simulink model "MalaksModel"  (R2022a)
settings: Solver=FixedStepAuto  StartTime=0.0  StopTime=10  FixedStep=0.001  MaxStep=1  MinStep=5e-4  RelTol=1e-3  EnableMultiTasking=on
values from neighbouring files (symbols this model uses):
  B = 0.00416    [Allan_Param.m]
  b1 = Bf/2    (= 0.776)    [model_10DOF_revised.m]
  b2 = b1    (= 0.776)    [model_10DOF_revised.m]
  b3 = Br/2    (= 0.78)    [model_10DOF_revised.m]
  b4 = b3    (= 0.78)    [model_10DOF_revised.m]
  Beq = 0.0001    [model_10DOF_revised.m]
  Bf = 1.552    [model_10DOF_revised.m]
  cs1 = 4500    [model_10DOF_revised.m]
  cs2 = 4500    [model_10DOF_revised.m]
  cs3 = 11207    [model_10DOF_revised.m]
  dpc = h-hzpc    (= 0.4878144918)    [model_10DOF_revised.m]
  drc = h-hzrc    (= 0.4878144918)    [model_10DOF_revised.m]
  Fs = 100    [Allan_Param.m]
  g = 9.81    [model_10DOF_revised.m]
  hzpc = 0.05    [model_10DOF_revised.m]
  hzrc = 0.05    [model_10DOF_revised.m]
  Ix = 233.072773102 + m*drc^2    (= 616.009936849)    [model_10DOF_revised.m]
  Ix_Iy = Ix -Iy    (= -852.927226898)    [model_10DOF_revised.m]
  Iy = 1086 + m*dpc^2    (= 1468.93716375)    [model_10DOF_revised.m]
  Iy_Iz = Iy -Iz    (= 281.937163747)    [model_10DOF_revised.m]
  Iz = 1187    [model_10DOF_revised.m]
  Iz_Ix = Iz -Ix    (= 570.990063151)    [model_10DOF_revised.m]
  Jeq = 0.00025    [model_10DOF_revised.m]
  K = 1.4e-3    (= 0.0014)    [Allan_Param.m]
  Ka = 0.05    [model_10DOF_revised.m]
  Ke = 0.168    [model_10DOF_revised.m]
  L = 2.72    [model_10DOF_revised.m]
  l1 = 1.12695753    [model_10DOF_revised.m]
  l2 = L-l1    (= 1.59304247)    [model_10DOF_revised.m]
  Leq = 1.5e-3    (= 0.0015)    [model_10DOF_revised.m]
  m = MT-(muf+mur)    (= 1609.23)    [model_10DOF_revised.m]
  mu = 0.8    [model_10DOF_revised.m]
  mu1 = muf/2    (= 49.5)    [model_10DOF_revised.m]
  mu2 = mu1    (= 49.5)    [model_10DOF_revised.m]
  mu3 = mur/2    (= 42)    [model_10DOF_revised.m]
  mu4 = mu3    (= 42)    [model_10DOF_revised.m]
  N = 0.00166667    [Allan_Param.m]
  radius = 40    [path1.m]
  Req = 0.5    [model_10DOF_revised.m]
  ro = 0    [Input.m]
  sw_delta_f = 1    [Input.m]
  Tc = 32    [Allan_Param.m]
  THETAo = 0    [Input.m]
  tpo = cp/6    (= 0.0333333333333)    [Input.m]
  vxo = 10    [Input.m]
  vyo = 0    [Input.m]
  Ws1 = (l2*Ws)/(2*L)    (= 4622.91152767)    [model_10DOF_revised.m]
  x = 0:1:200    [look_ahead.m]    (also in path1.m = x(:))
  Xo = 0    [Input.m]
  y = l_des    [look_ahead.m]    (also in path1.m = zeros(size(x)))
  Yo = 0    [Input.m]
  zu1_0 = -W1/k1t    (= -0.0255425326383)    [model_10DOF_revised.m]
  zu2_0 = -W2/k2t    (= -0.0255425326383)    [model_10DOF_revised.m]
  zu3_0 = -W3/k3t    (= -0.0184119081117)    [model_10DOF_revised.m]
  zu4_0 = -W4/k4t    (= -0.0184119081117)    [model_10DOF_revised.m]
undefined symbols (not defined in the file or in its folder): sw_phi, sw_psi, sw_theta, sw_x, sw_y, sw_zs, sw_zu1, sw_zu2, sw_zu3, sw_zu4
libraries: slpidlib x6, ec_arm_cortex_a_lib x1
(part 2 of 2)

== system MalaksModel/PID DC motor1/Ratchet ==
  d2 : Inport  OutDataTypeStr=double
  Memory3 : Memory
  Memory4 : Memory
  Ratchet : MATLAB Function  TreatAsAtomicUnit=on
  Switch : MATLAB Function  TreatAsAtomicUnit=on
  Theta : Outport  OutDataTypeStr=double
  wires:
  Memory3/1 -> Switch/2(d1)
  d2/1 -> Ratchet/1(d2), Switch/1(d2)
  Switch/2(d) -> Memory3/1
  Memory4/1 -> Ratchet/2(d1)
  Ratchet/1(y) -> Memory4/1, Theta/1  "Theta"
  Switch/1(y) -> Ratchet/3(s)

== system MalaksModel/PID DC motor2/Ratchet ==
  d2 : Inport  OutDataTypeStr=double
  Memory3 : Memory
  Memory4 : Memory
  Ratchet : MATLAB Function  TreatAsAtomicUnit=on
  Switch : MATLAB Function  TreatAsAtomicUnit=on
  Theta : Outport  OutDataTypeStr=double
  wires:
  Memory3/1 -> Switch/2(d1)
  d2/1 -> Ratchet/1(d2), Switch/1(d2)
  Switch/2(d) -> Memory3/1
  Memory4/1 -> Ratchet/2(d1)
  Ratchet/1(y) -> Memory4/1, Theta/1  "Theta"
  Switch/1(y) -> Ratchet/3(s)

== system MalaksModel/PID DC motor3/Ratchet ==
  d2 : Inport  OutDataTypeStr=double
  Memory3 : Memory
  Memory4 : Memory
  Ratchet : MATLAB Function  TreatAsAtomicUnit=on
  Switch : MATLAB Function  TreatAsAtomicUnit=on
  Theta : Outport  OutDataTypeStr=double
  wires:
  Memory3/1 -> Switch/2(d1)
  d2/1 -> Ratchet/1(d2), Switch/1(d2)
  Switch/2(d) -> Memory3/1
  Memory4/1 -> Ratchet/2(d1)
  Ratchet/1(y) -> Memory4/1, Theta/1  "Theta"
  Switch/1(y) -> Ratchet/3(s)

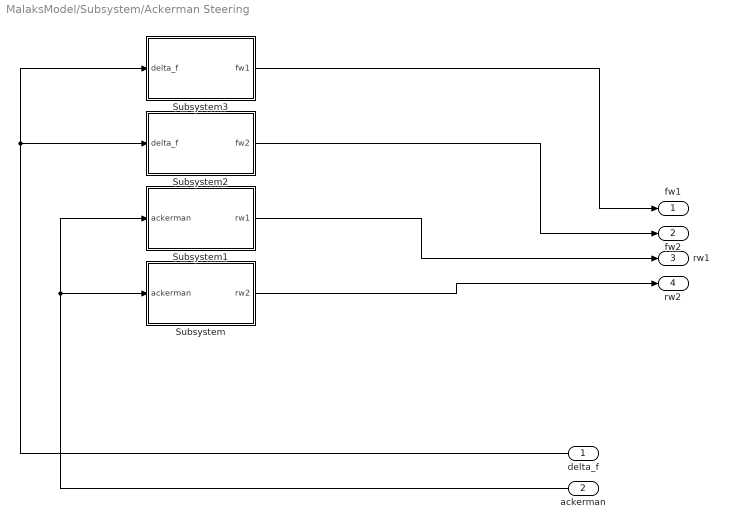
== system MalaksModel/Subsystem/Ackerman Steering ==
  delta_f : Inport  OutDataTypeStr=double
  ackerman : Inport  Port=2  OutDataTypeStr=double
  Subsystem : Subsystem
  Subsystem1 : Subsystem
  Subsystem2 : Subsystem
  Subsystem3 : Subsystem
  fw1 : Outport  OutDataTypeStr=double
  fw2 : Outport  Port=2  OutDataTypeStr=double
  rw1 : Outport  Port=3  OutDataTypeStr=double
  rw2 : Outport  Port=4  OutDataTypeStr=double
  wires:
  ackerman/1 -> Subsystem1/1(ackerman), Subsystem/1(ackerman)
  delta_f/1 -> Subsystem3/1(delta_f), Subsystem2/1(delta_f)
  Subsystem1/1(rw1) -> rw1/1
  Subsystem/1(rw2) -> rw2/1
  Subsystem3/1(fw1) -> fw1/1
  Subsystem2/1(fw2) -> fw2/1

== system MalaksModel/Subsystem/RWS ==
  delta_f : Inport  OutDataTypeStr=double
  vx : Inport  Port=2  OutDataTypeStr=double
  Constant : Constant  Value=l1
  Constant1 : Constant  Value=l2
  Constant2 : Constant  Value=L
  Constant3 : Constant  Value=m
  Constant4 : Constant  Value=cs3
  Constant5 : Constant  Value=cs2
  MATLAB Function : MATLAB Function  TreatAsAtomicUnit=on
  delta_r : Outport  OutDataTypeStr=double
  wires:
  Constant1/1 -> MATLAB Function/4(l2)
  vx/1 -> MATLAB Function/2(vx)
  Constant/1 -> MATLAB Function/3(l1)
  Constant3/1 -> MATLAB Function/6(m)
  Constant5/1 -> MATLAB Function/8(cs2)
  Constant2/1 -> MATLAB Function/5(L)
  Constant4/1 -> MATLAB Function/7(cs3)
  MATLAB Function/1(delta_r) -> delta_r/1
  delta_f/1 -> MATLAB Function/1(delta_f)

== system MalaksModel/Driver Steering Control/Subsystem/If Action Subsystem ==
  In1 : Inport
  Action Port : ActionPort  ActionPortLabel=if(u1 == 0)
  Out1 : Outport
  wires:
  In1/1 -> Out1/1

== system MalaksModel/Driver Steering Control/Subsystem/If Action Subsystem1 ==
  In1 : Inport
  Action Port : ActionPort  ActionPortLabel=elseif(u1 == 1)
  Out1 : Outport
  wires:
  In1/1 -> Out1/1

== system MalaksModel/Driver Steering Control/Subsystem1/If Action Subsystem ==
  In1 : Inport
  Action Port : ActionPort  ActionPortLabel=if(u1 == 0)
  Out1 : Outport
  wires:
  In1/1 -> Out1/1

== system MalaksModel/Driver Steering Control/Subsystem1/If Action Subsystem1 ==
  In1 : Inport
  Action Port : ActionPort  ActionPortLabel=elseif(u1 == 1)
  Out1 : Outport
  wires:
  In1/1 -> Out1/1

== system MalaksModel/Subsystem/Ackerman Steering/Subsystem ==
  ackerman : Inport
  Constant2 : Constant  Value=Bf
  Constant3 : Constant  Value=L
  MATLAB Function3 : MATLAB Function  TreatAsAtomicUnit=on
  rw2 : Outport
  wires:
  Constant3/1 -> MATLAB Function3/3(L)
  ackerman/1 -> MATLAB Function3/1(ackerman)
  Constant2/1 -> MATLAB Function3/2(Bf)
  MATLAB Function3/1(rw2) -> rw2/1

== system MalaksModel/Subsystem/Ackerman Steering/Subsystem1 ==
  ackerman : Inport
  Constant : Constant  Value=Bf
  Constant1 : Constant  Value=L
  MATLAB Function : MATLAB Function  TreatAsAtomicUnit=on
  rw1 : Outport
  wires:
  MATLAB Function/1(rw1) -> rw1/1
  Constant1/1 -> MATLAB Function/3(L)
  Constant/1 -> MATLAB Function/2(Bf)
  ackerman/1 -> MATLAB Function/1(ackerman)

== system MalaksModel/Subsystem/Ackerman Steering/Subsystem2 ==
  delta_f : Inport
  Constant6 : Constant  Value=Bf
  Constant7 : Constant  Value=L
  MATLAB Function5 : MATLAB Function  TreatAsAtomicUnit=on
  fw2 : Outport
  wires:
  MATLAB Function5/1(fw2) -> fw2/1
  Constant6/1 -> MATLAB Function5/2(Bf)
  Constant7/1 -> MATLAB Function5/3(L)
  delta_f/1 -> MATLAB Function5/1(delta_f)

== system MalaksModel/Subsystem/Ackerman Steering/Subsystem3 ==
  delta_f : Inport
  Constant4 : Constant  Value=Bf
  Constant5 : Constant  Value=L
  MATLAB Function4 : MATLAB Function  TreatAsAtomicUnit=on
  fw1 : Outport
  wires:
  Constant5/1 -> MATLAB Function4/3(L)
  delta_f/1 -> MATLAB Function4/1(delta_f)
  Constant4/1 -> MATLAB Function4/2(Bf)
  MATLAB Function4/1(fw1) -> fw1/1

== matlab function MalaksModel/Vehicle model/MATLAB Function ==
  data: y input size=[3 3]; Dz1 output; Dz2 output; Dz3 output; Dz4 output; l1 parameter; l2 parameter; b1 parameter; b2 parameter; b3 parameter; b4 parameter
function [Dz1,Dz2,Dz3, Dz4] = fcn(y,l1, l2, b1, b2, b3, b4)


Dz = y*[l1;-b1;0];
Dz1 = Dz(3);

Dz = y*[l1;b2;0];
Dz2 = Dz(3);

Dz = y*[-l2;-b3;0];
Dz3 = Dz(3);

Dz = y*[-l2;b4;0];
Dz4 = Dz(3);

== matlab function MalaksModel/Driver Steering Control/FWS Controller ==
  data: loc_act input; ackerman output size=1 [1..2]; vx input; C_alpha input size=1; x parameter; y parameter; m parameter; l2 parameter; l1 parameter; radius parameter
function ackerman = fcn(loc_act, vx, C_alpha, x, y, m, l2, l1, radius)

n = size(x,1); % number of points defined in path in workspace

%C_alpha = 100000;  % cornering stiffness      (N/rad) 

ld =9;   %look ahead distance
trans =[cos(loc_act(3)) sin(loc_act(3)); sin(loc_act(3)) -cos(loc_act(3))];% transformation matrix

if radius == 0
  radius = 1000;
end

Traj = cell(n,1);
Traj_loc = cell(n,1); 

 for i=1:1:n %trajectory defined in global frame
     Traj{i} = [x(i); y(i)];
 end

 for i=1:1:n    %trajectory defined in local frame
     Traj_loc{i} = trans*Traj{i};
 end

%----------------------------------------------------------------------------------------------------------------------
k=1:1:5;
x_ld = loc_act(1) +(k/5)*ld*cos(loc_act(3));
y_ld = loc_act(2) +(k/5)*ld*sin(loc_act(3));

PP = {[x_ld(1) ;y_ld(1)],[x_ld(2); y_ld(2)],[x_ld(3); y_ld(3)],[x_ld(4) ;y_ld(4)],[x_ld(5); y_ld(5)]};  
PP_loc = {[0 ;0],[0; 0],[0; 0],[0 ;0],[0; 0]};
%-----------------------------------------------------------------------------------------------------------------------

 for i=1:1:5   
     PP_loc{i} = trans*PP{i}; %PP defined in local frame
 end
%-----------------------------------------------------------------------------------------------------------------------
% Now we have both PP_loc and Traj_local defined in local frame, we can
% find offsets e(i) by finding the smallest x-difference between them

e_off = [0;0;0;0;0];
e_offi = [0;0;0;0;0];

for i=1:1:5
   err = 1000;
   for j=1:1:n
       ex = Traj_loc{j}(1)-PP_loc{i}(1);
       ey = Traj_loc{j}(2)-PP_loc{i}(2);
   
       if abs(ex)<err && abs(ey)< radius 
           err=abs(ex);
           
           e_off(i) = ex;
           e_offi(i) = Traj_loc{j}(2)-PP_loc{i}(2);
       end
   end
end 

%------------------------------------------------------------------------------------------------------------------------------
%G = [0.1 0.3 0.5 0.4 0.2 ];
%G = [0.1 0.2 0.5 0.4 0.3 ];

%G = [0.09 0.36 0.45 0.36 0.8 ];

%G = [0.4 1.2 2 1.6 0.8 ]; 
G = [0.2 0.6 1 0.8 0.4 ];

%G = [0.133 0.4 0.67 0.534 0.4 ];

sum=0;  

for n=1:1:5
    sum = sum+ e_offi(n)*G(n);  %  This is sum of product gains and offsets
end

T =  l2-(l1*m*vx^2)/(C_alpha*(l1+l2));

L = (2*(l1+l2-(m*vx^2*(l1*C_alpha-l2*C_alpha))/((l1+l2)*C_alpha*C_alpha)) / (ld*(ld+2*T)));

ackerman=(-L*sum)*16; % this is the ackerman steering angle, which is (lmadao+lamdai0/2

== matlab function MalaksModel/Driver Throttle Control/MATLAB Function ==
  data: u input; kpf output; kdf output; kif output
function [kpf,kdf,kif] = fcn(u)
kp=70;
ki=0.05;
kd=0.05;
kpf=kp*u+5;
kif=ki*u;
kdf=kd*u;

== matlab function MalaksModel/Subsystem/RWS/MATLAB Function ==
  data: delta_f input; delta_r output; vx input; l1 input; l2 input; L input; m input; cs3 input; cs2 input
function delta_r = fcn(delta_f,vx,l1,l2,L,m,cs3,cs2)

delta_r=delta_f*((-l2+((m*l1)/(cs3*L))*vx^2)/((l1+((m*l2)/(cs2*L))*vx^2)));

== matlab function MalaksModel/Subsystem/Ackerman Steering/Subsystem1/MATLAB Function ==
  data: ackerman input; rw1 output; Bf input; L input
function rw1  = fcn(ackerman, Bf, L)



rw1 = atan((2*L*sin(ackerman))/(2*L*cos(ackerman)-Bf*sin(ackerman)));

== matlab function MalaksModel/Subsystem/Ackerman Steering/Subsystem/MATLAB Function3 ==
  data: ackerman input; rw2 output; Bf input; L input
function rw2  = fcn(ackerman, Bf, L)




rw2 = atan((2*L*sin(ackerman))/(2*L*cos(ackerman)+Bf*sin(ackerman)));

== matlab function MalaksModel/PID DC motor/MATLAB Function ==
  data: Fx input; rt output; Fy input; tp input
function rt = fcn(Fx,Fy,tp)

rt=Fx*0.15+Fy*tp;

== matlab function MalaksModel/PID DC motor/Ratchet/Ratchet ==
  data: d2 input double; d1 input double; y output double; s input double
function y = fcn(d2,d1,s)
if s==1
    if d2>d1
    y=d2;
        else
    y=d1;
    end
else 

    if d1>d2
        y=d2;
    else
        y=d1;
    end


end

== matlab function MalaksModel/Subsystem/Ackerman Steering/Subsystem3/MATLAB Function4 ==
  data: delta_f input; fw1 output; Bf input; L input
function fw1  = fcn(delta_f, Bf, L)


fw1 = atan((2*L*sin(delta_f))/(2*L*cos(delta_f)-Bf*sin(delta_f)));

== matlab function MalaksModel/Subsystem/Ackerman Steering/Subsystem2/MATLAB Function5 ==
  data: delta_f input; fw2 output; Bf input; L input
function fw2  = fcn(delta_f, Bf, L)




fw2 = atan((2*L*sin(delta_f))/(2*L*cos(delta_f)+Bf*sin(delta_f)));

== matlab function MalaksModel/Orientation Gyro/Allan Noise/MATLAB Function ==
  data: Fs input; Phi output; N input; K input; B input; Tc input; Qbk output; Qkk output; Qnk output
function [Phi,Qbk,Qkk,Qnk] = fcn(Fs,N,K,B,Tc)
Sn=N^2;
Sk=K^2;
mu_b=1/Tc; 
Sb=(2*B^2*log(2))/(pi*0.4365^2*Tc);

A_t=[-mu_b 0;
    0 0];
B_t=[1 0;
    0 1];


S_w_z=[Sb 0;
        0 Sk];
A_c=[0 0 0 0; 0 0 0 0; 0 0 0 0; 0 0 0 0];
A_c(1:2,1:2) = -1*A_t;
A_c(1:2,3:4) = B_t * S_w_z * B_t';
A_c(3:4,3:4) = A_t';

A_c=A_c*1/Fs;
B_c=expm(A_c);

Phi=B_c(3:4,3:4);

% From eqn. (4.116) of [3]
Qd=B_c(1:2,3:4);

% Discrete time bias instability driving noise
Qbk=Qd(1,1);

% Discsrete time rate random walk process noise
Qkk=Qd(2,2);

% Discsrete time random walk process noise
% See IEEE CSM eqn. (62)
Qnk=Sn*Fs;

== matlab function MalaksModel/Orientation Gyro/Allan Noise/MATLAB Function1 ==
  settings: updateMethod=DISCRETE
  data: Phi input double; Z output double; Qbk input double; Qkk input double; Qnk input double; t input double; Fs input double; Z_b1 input double; Z_b1 output; Z_b2 input double; Z_b2 output
function [Z,Z_b1,Z_b2]= fcn(Phi, Qbk, Qkk, Qnk, t,Fs,Z_b1, Z_b2)
Z_b=[Z_b1;Z_b2];
if mod(t,1/Fs)==0
    sQbk = sqrt(Qbk);
    sQkk = sqrt(Qkk);
    sQnk = sqrt(Qnk);      
%     Z    = zeros(L_n,1);

    n_b = sQbk * randn(1,1);
    n_k = sQkk * randn(1,1);
    n_n = sQnk * randn(1,1);

    Z_b = Phi*Z_b + [n_b;n_k];
    Z_b1=Z_b(1);
    Z_b2=Z_b(2);
    Z= [1 1] * Z_b + n_n;
else
    Z=0;
    Z_b1=double(Z_b1);
    Z_b2=double(Z_b2);

end

== matlab function MalaksModel/PID DC motor/pneumatic trail  ==
  data: tpo input; tp output; cs1 input; mu input; Fz input; alpha input
function tp = fcn(tpo, cs1, mu, Fz, alpha)

I_f=1/(mu*Fz);
alpha_sl=atan(3/(cs1*I_f));

if abs(alpha) <= alpha_sl
    tp=tpo-(tpo*cs1*I_f*tan(alpha)/3);
else
    tp=0;
end

== matlab function MalaksModel/PID DC motor/Ratchet/Switch ==
  data: d2 input double; d1 input double; y output double; d output double
function [y,d] = fcn(d2,d1)

if d2>d1
    y=1;
else
    y=0;
end
d=d2;

== matlab function MalaksModel/PID DC motor1/MATLAB Function ==
  data: Fx input; rt output; Fy input; tp input
function rt = fcn(Fx,Fy,tp)

rt=Fx*0.15+Fy*tp;

== matlab function MalaksModel/PID DC motor1/Ratchet/Ratchet ==
  data: d2 input double; d1 input double; y output double; s input double
function y = fcn(d2,d1,s)
if s==1
    if d2>d1
    y=d2;
        else
    y=d1;
    end
else 

    if d1>d2
        y=d2;
    else
        y=d1;
    end


end

== matlab function MalaksModel/PID DC motor1/Ratchet/Switch ==
  data: d2 input double; d1 input double; y output double; d output double
function [y,d] = fcn(d2,d1)

if d2>d1
    y=1;
else
    y=0;
end
d=d2;

== matlab function MalaksModel/PID DC motor1/pneumatic trail  ==
  data: tpo input; tp output; cs1 input; mu input; Fz input; alpha input
function tp = fcn(tpo, cs1, mu, Fz, alpha)

I_f=1/(mu*Fz);
alpha_sl=atan(3/(cs1*I_f));

if abs(alpha) <= alpha_sl
    tp=tpo-(tpo*cs1*I_f*tan(alpha)/3);
else
    tp=0;
end

== matlab function MalaksModel/PID DC motor2/MATLAB Function ==
  data: Fx input; rt output; Fy input; tp input
function rt = fcn(Fx,Fy,tp)

rt=Fx*0.15+Fy*tp;

== matlab function MalaksModel/PID DC motor2/Ratchet/Ratchet ==
  data: d2 input double; d1 input double; y output double; s input double
function y = fcn(d2,d1,s)
if s==1
    if d2>d1
    y=d2;
        else
    y=d1;
    end
else 

    if d1>d2
        y=d2;
    else
        y=d1;
    end


end

== matlab function MalaksModel/PID DC motor2/Ratchet/Switch ==
  data: d2 input double; d1 input double; y output double; d output double
function [y,d] = fcn(d2,d1)

if d2>d1
    y=1;
else
    y=0;
end
d=d2;

== matlab function MalaksModel/PID DC motor2/pneumatic trail  ==
  data: tpo input; tp output; cs1 input; mu input; Fz input; alpha input
function tp = fcn(tpo, cs1, mu, Fz, alpha)

I_f=1/(mu*Fz);
alpha_sl=atan(3/(cs1*I_f));

if abs(alpha) <= alpha_sl
    tp=tpo-(tpo*cs1*I_f*tan(alpha)/3);
else
    tp=0;
end

== matlab function MalaksModel/Vehicle model/MATLAB Function1 ==
  data: lamda input; alpha output size=[4 1]; r input; vx input; vy input; l1 parameter; l2 parameter
function alpha  = fcn(lamda,r,vx,vy, l1, l2)

alpha1 = lamda(1) -((vy+l1*r)/vx);
alpha2 = lamda(2) -((vy+l1*r)/vx);
alpha3 = lamda(3) -((vy-l2*r)/vx);
alpha4 = lamda(4) -((vy-l2*r)/vx);


alpha = [alpha1; alpha2; alpha3; alpha4];

== matlab function MalaksModel/PID DC motor3/MATLAB Function ==
  data: Fx input double; rt output double; Fy input double; tp input double
function rt = fcn(Fx,Fy,tp)

rt=Fx*0.15+Fy*tp;

== matlab function MalaksModel/PID DC motor3/Ratchet/Ratchet ==
  data: d2 input double; d1 input double; y output double; s input double
function y = fcn(d2,d1,s)
if s==1
    if d2>d1
    y=d2;
        else
    y=d1;
    end
else 

    if d1>d2
        y=d2;
    else
        y=d1;
    end


end

== matlab function MalaksModel/PID DC motor3/Ratchet/Switch ==
  data: d2 input double; d1 input double; y output double; d output double
function [y,d] = fcn(d2,d1)

if d2>d1
    y=1;
else
    y=0;
end
d=d2;

== matlab function MalaksModel/PID DC motor3/pneumatic trail  ==
  data: tpo input; tp output; cs1 input; mu input; Fz input; alpha input
function tp = fcn(tpo, cs1, mu, Fz, alpha)

I_f=1/(mu*Fz);
alpha_sl=atan(3/(cs1*I_f));

if abs(alpha) <= alpha_sl
    tp=tpo-(tpo*cs1*I_f*tan(alpha)/3);
else
    tp=0;
end

== matlab function MalaksModel/MATLAB Function ==
  data: t input; u input; y output
function y = fcn(t,u)

if t>9.9
    y=0;
else
    y=u;
end

== matlab function MalaksModel/Vehicle model/MATLAB Function4 ==
  data: Fs output size=[4 1]; Ft output size=[4,1]; zs input; zs_dot input; Dz1 input; Dz1_dot input; Dz2 input; Dz2_dot input; Dz3 input; Dz3_dot input; Dz4 input; Dz4_dot input; zu3 input; zu3_dot input; zu4 input; zu4_dot input; zu1 input; zu1_dot input; zu2 input; zu2_dot input
function [Fs,Ft]  = fcn(zs,zs_dot,Dz1, Dz1_dot,Dz2,Dz2_dot,Dz3, Dz3_dot, Dz4, Dz4_dot, zu3, zu3_dot, zu4, zu4_dot, zu1, zu1_dot,zu2, zu2_dot)

%Fs = [0;0;0;0];
%Ft = [0;0;0;0];


ks1 =265000 ;  % wheel rate (Calculated from Adams)
ks2 =265000;
ks3 =52500 ;
ks4 =52500 ;

cs1 =4500 ;     % obtained from Adams
cs2 =4500  ;
cs3 =11207  ;
cs4 =11207  ;

k1t = 200000;
k2t = 200000;
k3t = 200000;
k4t = 200000;


Fs1 = ks1*(zs - Dz1 - zu1)+ cs1*(zs_dot - Dz1_dot -zu1_dot);
Fs2 = ks2*(zs - Dz2 - zu2)+ cs2*(zs_dot - Dz2_dot -zu2_dot); 
Fs3 = ks3*(zs - Dz3 - zu3)+ cs3*(zs_dot - Dz3_dot -zu3_dot);
Fs4 = ks4*(zs - Dz4 - zu4)+ cs4*(zs_dot - Dz4_dot -zu4_dot);

% Fs1 = ks1*(zs - zu1)+ cs1*(zs_dot - Dz1_dot -zu1_dot);
% Fs2 = ks2*(zs - zu2)+ cs2*(zs_dot - Dz2_dot -zu2_dot); 
% Fs3 = ks3*(zs - zu3)+ cs3*(zs_dot - Dz3_dot -zu3_dot);
% Fs4 = ks4*(zs - zu4)+ cs4*(zs_dot - Dz4_dot -zu4_dot);

Ft1 = k1t*(zu1);
Ft2 = k2t*(zu2);
Ft3 = k3t*(zu3);
Ft4 = k4t*(zu4);

Fs = -[Fs1;Fs2;Fs3;Fs4];
Ft = -[Ft1;Ft2; Ft3; Ft4];

== matlab function MalaksModel/Vehicle model/MATLAB Function2 ==
  data: alpha input; Fy output; Fz input; C_alpha_f output size=1; Model parameter
function [Fy, C_alpha_f] = fcn(alpha, Fz, Model)

Fz=Fz./1000;

a0 = 1.3;
a1 = -22.1;
a2 = 1011;
a3 = 1078;
a4 = 1.82;
a5 = 0.208;
a6 = 0;
a7 = -0.354;
a8 = 0.707;

C=[a0;a0;a0;a0];
D = (a1.*Fz.^2)+(a2.*Fz);
BCD = a3*sin(a4*atan(a5.*Fz));

C_alpha = [0;0;0;0];

C_alpha(3) = (BCD(3)+BCD(4))*57.3;
C_alpha(4) = (BCD(3)+BCD(4))*57.3;
C_alpha(2) = (BCD(1)+BCD(2))*57.3;
C_alpha(1) = (BCD(1)+BCD(2))*57.3;

C_alpha_f = C_alpha(1);

B = BCD./(C.*D);
E = (a6.*Fz.^2)+(a7.*Fz)+ a8;

S = ((ones(4,1)-E)*57.3.*alpha) + ((E./B).*atan(B.*57.3.*alpha));

Fy = [0;0;0;0];

if Model == 1
Fy(1) = C_alpha(1)*alpha(1);
Fy(2) = C_alpha(2)*alpha(2);
Fy(3) = C_alpha(3)*alpha(3);
Fy(4) = C_alpha(4)*alpha(4);
    
else
Fy=D.*sin(C.*atan(B.*S));
end

== matlab function MalaksModel/Vehicle model/MATLAB Function3 ==
  data: phi input; y output size=[3 3]; theta input; psi input
function y = fcn(phi,theta,psi)

y = [cos(theta)*cos(psi) cos(phi)*sin(psi)+sin(phi)*sin(theta)*cos(psi) sin(phi)*sin(psi)-cos(phi)*sin(theta)*cos(psi);
    
    -cos(theta)*sin(psi) cos(phi)*cos(psi)-sin(phi)*sin(theta)*sin(psi) sin(phi)*cos(psi)+cos(phi)*sin(theta)*sin(psi);
    
    sin(theta)       -sin(phi)*cos(theta)        cos(phi)*cos(theta)

    ];

y=inv(y);

== matlab function MalaksModel/Vehicle model/MATLAB Function5 ==
  data: theta_dot input; euler_dot1 output; phi_dot input; psi_dot input; euler1 input; euler2 input; euler3 input; euler_dot2 output; euler_dot3 output
function [euler_dot1, euler_dot2, euler_dot3] = fcn(theta_dot,phi_dot,psi_dot, euler1,euler2,euler3)

euler_dot1 = (cos(euler3)*phi_dot - sin(euler3)*theta_dot)/cos(euler2);
euler_dot2 = sin(euler3)*phi_dot + cos(euler3)*theta_dot;
euler_dot3 = (sin(euler3)*theta_dot - cos(euler3)*phi_dot)*tan(theta_dot) + psi_dot;

%euler_dot1 = [euler1_dot;euler2_dot;euler3_dot];
